simulink model "F16_fcs111"  (Simulink 9.1)
settings: Solver=ode3  StartTime=0.0  StopTime=simtime  FixedStep=0.001  RelTol=1e-3  EnableMultiTasking=on
values from neighbouring files (symbols this model uses):
  alpha_trim = xu(3)    [runF16fcs.m]
  dlef_trim = uu(5)    [runF16fcs.m]
  fi_flag_Simulink = 1    [runF16fcs.m]
  V_trim = xu(1)    [runF16fcs.m]
undefined symbols (not defined in the file or in its folder): Earth, m, s, WGS84
libraries: simulink_extras x6, aerolibconvert2 x2, sharedtransform x2, aerolibtransform2 x1, aerolibconvert x1, aerolibobsolete x1, aerolibanimutils x1
settings Model: SuppressorTable="22 serialization::archive 11 0 6 0 0 1 8 0 0 0 0 6 0 0 1 0 49 F16_fcs111/Display Results/cascvt/Unit Conversion 0 6 0 0 1 8 0 0 0 0 6 49 SimulinkFixedPoint:util:fxpParameterPrecisionLoss 0 0 0 6 0  11 Wenchao Lei 0 0 0 0 8 20180715 0 0 0 16 3 53 0 0"  Creator=larssonneveldt  LastModifiedBy=Wenchao Lei
settings DataIOCC: LimitDataPoints=on  SignalLoggingSaveFormat=ModelDataLogs  SignalLoggingName=sigsOut
settings OptimizationCC: ExpressionDepthLimit=2147483647  InitFltsAndDblsToZero=on
settings DebuggingCC: SignalResolutionControl=TryResolveAllWithWarning  MultiTaskDSMMsg=warning  MultiTaskCondExecSysMsg=none  ParameterPrecisionLossMsg=none  FcnCallInpInsideContextMsg=warning  StateNameClashWarn=warning
settings HardwareCC: TargetHWDeviceType=32-bit Generic  TargetUnknown=on  ProdEqTarget=off
settings GRTTargetCC: TargetFcnLib=ansi_tfl_tmw.mat

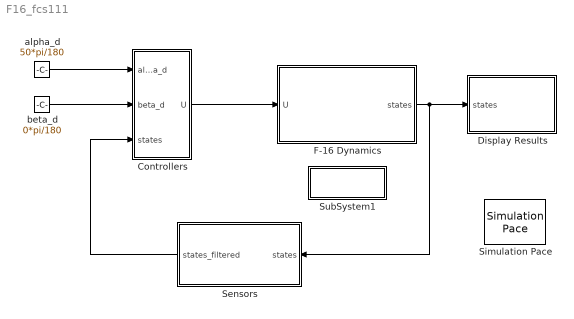
== system F16_fcs111 ==
  Controllers : Subsystem
  Display Results : Subsystem
  F-16 Dynamics : Subsystem
      mask Display: image(imread('aerodata/f16.jpg'))
  Sensors : Subsystem
  Simulation Pace : aerolibanimutils/Simulation Pace  SimulationPace=10  SleepMode=MATLAB Thread  OutputPaceError=off  SampleTime=-1
      settings: AttributesFormatString=%<SimulationPace> sec/sec
  SubSystem1 : Subsystem
      settings: OpenFcn=edit(fullfile(cd,'F16_dyn.c'))
      mask Display: disp('F16_dyn.c');
  alpha_d : Constant  Value=50*pi/180
  beta_d : Constant  Value=0*pi/180
  wires:
  F-16 Dynamics/1(states) -> Display Results/1(states), Sensors/1(states)
  Sensors/1(states_filtered) -> Controllers/3(states)
  beta_d/1 -> Controllers/2(beta_d)
  Controllers/1(U) -> F-16 Dynamics/1(U)
  alpha_d/1 -> Controllers/1(alpha_d)

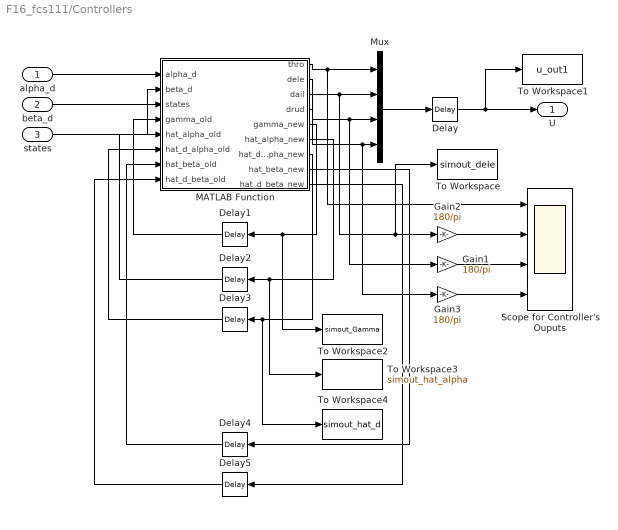
== system F16_fcs111/Controllers ==
  alpha_d : Inport
  beta_d : Inport  Port=2
  states : Inport  Port=3
  Delay : TransportDelay  DelayTime=0.02
  Delay1 : TransportDelay  DelayTime=0.01  InitialOutput=0.1*ones(3,1)
  Delay{2..5} (4 alike) : TransportDelay  DelayTime=0.01
  Gain1 : Gain  Gain=180/pi
  Gain2 : Gain  Gain=180/pi
  Gain3 : Gain  Gain=180/pi
  MATLAB Function : MATLAB Function  TreatAsAtomicUnit=on
  Mux : Mux
  Scope for Controller's Ouputs : Scope  NumInputPorts=4
  To Workspace : ToWorkspace  VariableName=simout_dele  SaveFormat=Structure With Time  SampleTime=-1
  To Workspace1 : ToWorkspace  VariableName=u_out1  SaveFormat=Structure With Time  SampleTime=-1
  To Workspace2 : ToWorkspace  VariableName=simout_Gamma  SaveFormat=Structure With Time  SampleTime=-1
  To Workspace3 : ToWorkspace  VariableName=simout_hat_alpha  SaveFormat=Structure With Time  SampleTime=-1
  To Workspace4 : ToWorkspace  VariableName=simout_hat_d  SaveFormat=Structure With Time  SampleTime=-1
  U : Outport
  wires:
  beta_d/1 -> MATLAB Function/2(beta_d)
  Mux/1 -> Delay/1
  Delay/1 -> U/1, To Workspace1/1
  states/1 -> MATLAB Function/3(states)
  alpha_d/1 -> MATLAB Function/1(alpha_d)
  Gain2/1 -> Scope for Controller's Ouputs/2
  Gain1/1 -> Scope for Controller's Ouputs/3
  Gain3/1 -> Scope for Controller's Ouputs/4
  Delay1/1 -> MATLAB Function/4(gamma_old)
  MATLAB Function/1(thro) -> Scope for Controller's Ouputs/1, Mux/1
  MATLAB Function/2(dele) -> To Workspace/1, Gain2/1, Mux/2
  MATLAB Function/3(dail) -> Gain1/1, Mux/3
  MATLAB Function/5(gamma_new) -> To Workspace2/1, Delay1/1
  MATLAB Function/4(drud) -> Gain3/1, Mux/4
  MATLAB Function/6(hat_alpha_new) -> To Workspace3/1, Delay2/1
  Delay2/1 -> MATLAB Function/5(hat_alpha_old)
  MATLAB Function/7(hat_d_alpha_new) -> To Workspace4/1, Delay3/1
  Delay3/1 -> MATLAB Function/6(hat_d_alpha_old)
  MATLAB Function/8(hat_beta_new) -> Delay4/1
  Delay4/1 -> MATLAB Function/7(hat_beta_old)
  MATLAB Function/9(hat_d_beta_new) -> Delay5/1
  Delay5/1 -> MATLAB Function/8(hat_d_beta_old)

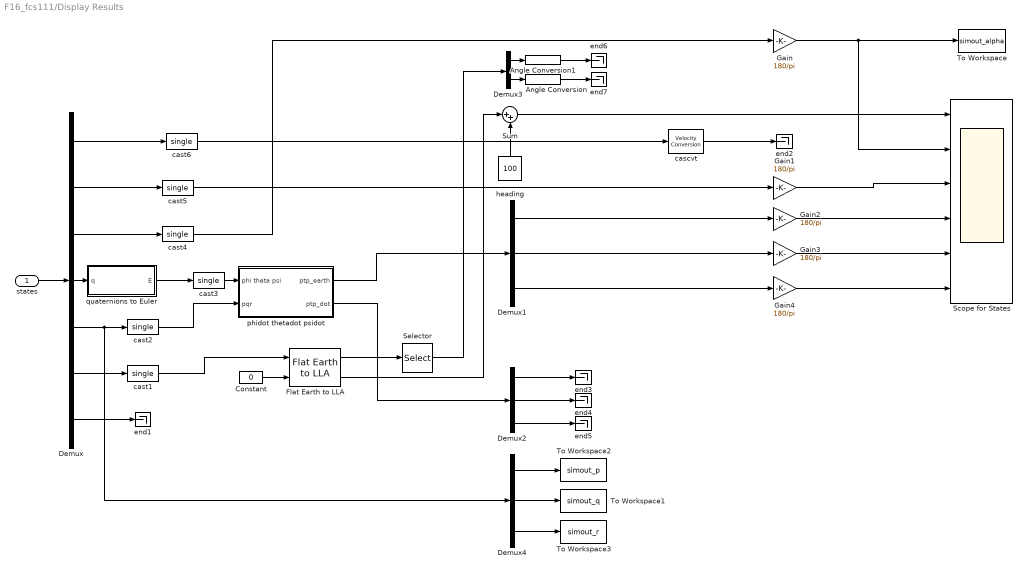
== system F16_fcs111/Display Results ==
  states : Inport
  Angle Conversion : aerolibconvert2/Angle Conversion  IU=deg  OU=rad
  Angle Conversion1 : aerolibconvert2/Angle Conversion  IU=deg  OU=rad
  Constant : Constant  Value=0
  Demux : Demux  Outputs=[1 1 1 4 3 3 3]
  Demux1 : Demux  Outputs=3
  Demux2 : Demux  Outputs=3
  Demux3 : Demux  Outputs=2
  Demux4 : Demux  Outputs=3
  Flat Earth to LLA : aerolibtransform2/Flat Earth to LLA  units=Metric (MKS)  ptype=Earth (WGS84)  F=1/298.257223563  R=6378137  LL0=[37.7889 -122.4778]  psi=0
  Gain{,1..4} (5 alike) : Gain  Gain=180/pi
  Scope for States : Scope  NumInputPorts=6
  Selector : Selector  InputPortWidth=2  IndexOptions=Index vector (dialog)  Indices=[2 1]  OutputSizes=1
  Sum : Sum  Inputs=|++
  To Workspace : ToWorkspace  VariableName=simout_alpha  SaveFormat=Structure With Time  SampleTime=-1
  To Workspace1 : ToWorkspace  VariableName=simout_q  SaveFormat=Structure With Time  SampleTime=-1
  To Workspace2 : ToWorkspace  VariableName=simout_p  SaveFormat=Structure With Time  SampleTime=-1
  To Workspace3 : ToWorkspace  VariableName=simout_r  SaveFormat=Structure With Time  SampleTime=-1
  cascvt : aerolibconvert/Velocity Conversion  IU=m/s  OU=kts
      settings: SourceProductName=Aerospace Blockset  SourceProductBaseCode=AE
  cast{1..6} (6 alike) : DataTypeConversion  OutDataTypeStr=single  SaturateOnIntegerOverflow=on
  end{1..7} (7 alike) : Terminator
  heading : Constant  Value=100
  phidot thetadot psidot : Subsystem
  quaternions to Euler : Subsystem
  wires:
  states/1 -> Demux/1
  Demux/1 -> cast6/1
  Demux/2 -> cast5/1
  Demux1/1 -> Gain2/1
  Demux1/3 -> Gain4/1
  Demux/3 -> cast4/1
  Demux/5 -> cast2/1, Demux4/1
  phidot thetadot psidot/1(ptp_earth) -> Demux1/1
  phidot thetadot psidot/2(ptp_dot) -> Demux2/1
  Demux/6 -> cast1/1
  Constant/1 -> Flat Earth to LLA/2
  Flat Earth to LLA/1 -> Selector/1
  Selector/1 -> Demux3/1
  Demux3/1 -> Angle Conversion1/1
  Demux3/2 -> Angle Conversion/1
  cast1/1 -> Flat Earth to LLA/1
  cast2/1 -> phidot thetadot psidot/2(pqr)
  cast3/1 -> phidot thetadot psidot/1(phi theta psi)
  cast4/1 -> Gain/1
  cast5/1 -> Gain1/1
  cast6/1 -> cascvt/1
  Flat Earth to LLA/2 -> Sum/1
  Sum/1 -> Scope for States/1
  heading/1 -> Sum/2
  quaternions to Euler/1(E) -> cast3/1
  Demux/4 -> quaternions to Euler/1(q)
  Demux/7 -> end1/1
  Gain3/1 -> Scope for States/5
  Gain2/1 -> Scope for States/4
  Gain4/1 -> Scope for States/6
  Demux1/2 -> Gain3/1
  Gain/1 -> Scope for States/2, To Workspace/1
  Gain1/1 -> Scope for States/3
  Demux4/1 -> To Workspace2/1
  Demux4/3 -> To Workspace3/1
  Demux4/2 -> To Workspace1/1
  cascvt/1 -> end2/1
  Demux2/1 -> end3/1
  Demux2/2 -> end4/1
  Demux2/3 -> end5/1
  Angle Conversion1/1 -> end6/1
  Angle Conversion/1 -> end7/1

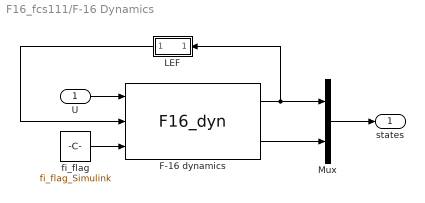
== system F16_fcs111/F-16 Dynamics ==
  U : Inport
  F-16 dynamics : S-Function  FunctionName=F16_dyn  Parameters=init_x  SFunctionDeploymentMode=off  EnableBusSupport=off
      mask Display: image(imread('aerodata/f16.jpg'))
  LEF : Subsystem
      mask Display: port_label('output', 1, 'dlef')
  Mux : Mux  Inputs=2
  fi_flag : Constant  Value=fi_flag_Simulink
  states : Outport
  wires:
  fi_flag/1 -> F-16 dynamics/3
  LEF/1("delta_lef ") -> F-16 dynamics/2
  U/1 -> F-16 dynamics/1
  F-16 dynamics/1 -> LEF/1(state), Mux/1
  F-16 dynamics/2 -> Mux/2
  Mux/1 -> states/1

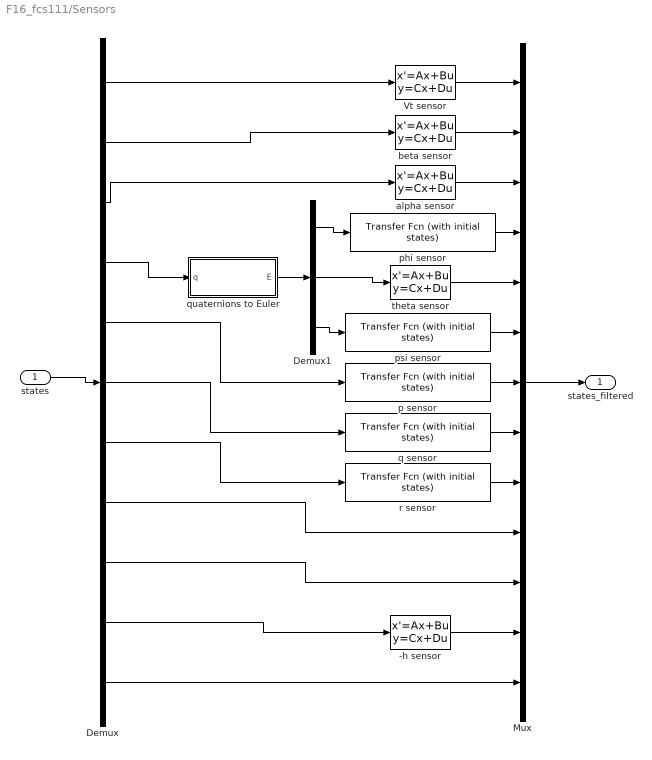
== system F16_fcs111/Sensors ==
  states : Inport
  -h sensor : StateSpace  A=-50  B=50  D=0  InitialCondition=alpha_trim
  Demux : Demux  Outputs=[ones(1,3) 4 ones(1,6) 3]
  Demux1 : Demux  Outputs=3
  Mux : Mux  Inputs=[ones(1,12) 3]
  Vt sensor : StateSpace  A=-50  B=50  D=0  InitialCondition=V_trim
  alpha sensor : StateSpace  A=-50  B=50  D=0  InitialCondition=alpha_trim
  beta sensor : StateSpace  A=-50  B=50  D=0  InitialCondition=0
  p sensor : simulink_extras/Additional Linear/Transfer Fcn (with initial states)  N=[0.0001903 0.005346 1]  D=[0.0004942 0.03082 1]  X0=[0 0]
  phi sensor : simulink_extras/Additional Linear/Transfer Fcn (with initial states)  N=[1]  D=[0.00104 0.0323 1]  X0=[0 0]
  psi sensor : simulink_extras/Additional Linear/Transfer Fcn (with initial states)  N=[1]  D=[0.00104 0.0323 1]  X0=[0 0]
  q sensor : simulink_extras/Additional Linear/Transfer Fcn (with initial states)  N=[0.0001903 0.005346 1]  D=[0.0004942 0.03082 1]  X0=[0 0]
  quaternions to Euler : Subsystem
  r sensor : simulink_extras/Additional Linear/Transfer Fcn (with initial states)  N=[0.0001903 0.005346 1]  D=[0.0004942 0.03082 1]  X0=[0 0]
  theta sensor : StateSpace  A=-50  B=50  D=0  InitialCondition=alpha_trim
  states_filtered : Outport
  wires:
  Mux/1 -> states_filtered/1
  states/1 -> Demux/1
  r sensor/1 -> Mux/9
  q sensor/1 -> Mux/8
  p sensor/1 -> Mux/7
  psi sensor/1 -> Mux/6
  phi sensor/1 -> Mux/4
  alpha sensor/1 -> Mux/3
  beta sensor/1 -> Mux/2
  Vt sensor/1 -> Mux/1
  Demux1/1 -> phi sensor/1
  Demux1/2 -> theta sensor/1
  Demux1/3 -> psi sensor/1
  -h sensor/1 -> Mux/12
  quaternions to Euler/1(E) -> Demux1/1
  theta sensor/1 -> Mux/5
  Demux/1 -> Vt sensor/1
  Demux/2 -> beta sensor/1
  Demux/3 -> alpha sensor/1
  Demux/4 -> quaternions to Euler/1(q)
  Demux/5 -> p sensor/1
  Demux/6 -> q sensor/1
  Demux/7 -> r sensor/1
  Demux/8 -> Mux/10
  Demux/9 -> Mux/11
  Demux/10 -> -h sensor/1
  Demux/11 -> Mux/13

== system F16_fcs111/SubSystem1 ==

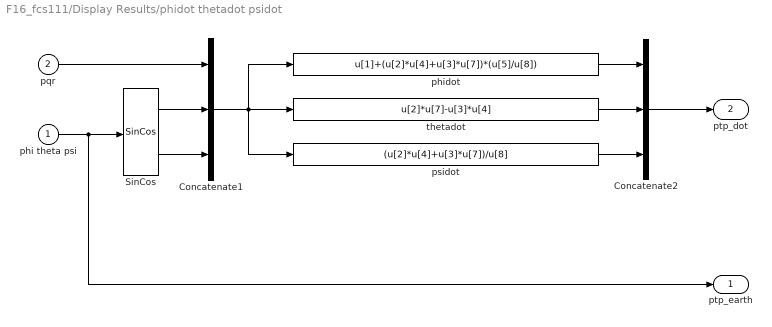
== system F16_fcs111/Display Results/phidot thetadot psidot ==
  phi theta psi : Inport
  pqr : Inport  Port=2
  Concatenate1 : Concatenate  NumInputs=3
  Concatenate2 : Concatenate  NumInputs=3
  SinCos : aerolibobsolete/SinCos
      settings: SourceProductName=Aerospace Blockset  SourceProductBaseCode=AE
  phidot : Fcn  Expr=u[1]+(u[2]*u[4]+u[3]*u[7])*(u[5]/u[8])
  psidot : Fcn  Expr=(u[2]*u[4]+u[3]*u[7])/u[8]
  thetadot : Fcn  Expr=u[2]*u[7]-u[3]*u[4]
  ptp_earth : Outport
  ptp_dot : Outport  Port=2
  wires:
  Concatenate1/1 -> psidot/1, phidot/1, thetadot/1
  pqr/1 -> Concatenate1/1
  phi theta psi/1 -> SinCos/1, ptp_earth/1
  psidot/1 -> Concatenate2/3
  thetadot/1 -> Concatenate2/2
  phidot/1 -> Concatenate2/1
  Concatenate2/1 -> ptp_dot/1
  SinCos/1 -> Concatenate1/2
  SinCos/2 -> Concatenate1/3

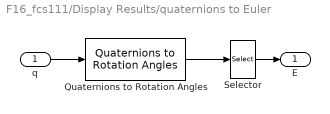
== system F16_fcs111/Display Results/quaternions to Euler ==
  q : Inport
  Quaternions to Rotation Angles : sharedtransform/Quaternions to Rotation Angles  rotationOrder=ZYX  aMode=aMode
      settings: SourceProductBaseCode=AE
  Selector : Selector  InputPortWidth=3  IndexOptions=Index vector (dialog)  Indices=[3 2 1]  OutputSizes=1
  E : Outport
  wires:
  Quaternions to Rotation Angles/1 -> Selector/1
  q/1 -> Quaternions to Rotation Angles/1
  Selector/1 -> E/1

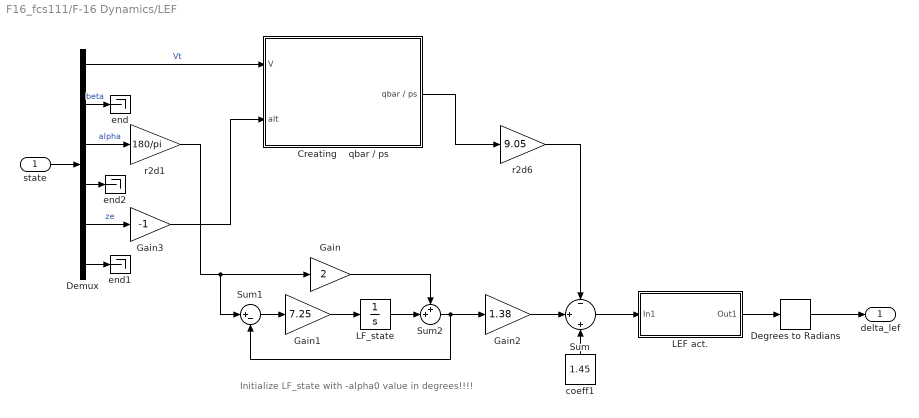
== system F16_fcs111/F-16 Dynamics/LEF ==
  note: Initialize LF_state with -alpha0 value in degrees!!!!
  state : Inport
  Creating    qbar / ps : Subsystem
  Degrees to Radians : simulink_extras/Transformations/Degrees to Radians
  Demux : Demux  Outputs=[1 1 1 9 1 1]
  Gain : Gain  Gain=2  SaturateOnIntegerOverflow=on  OutDataTypeStr=Inherit: Same as input  ParamDataTypeStr=Inherit: Same as input
  Gain1 : Gain  Gain=7.25  SaturateOnIntegerOverflow=on  OutDataTypeStr=Inherit: Same as input  ParamDataTypeStr=Inherit: Same as input
  Gain2 : Gain  Gain=1.38  SaturateOnIntegerOverflow=on  OutDataTypeStr=Inherit: Same as input  ParamDataTypeStr=Inherit: Same as input
  Gain3 : Gain  Gain=-1  SaturateOnIntegerOverflow=on  OutDataTypeStr=Inherit: Same as input  ParamDataTypeStr=Inherit: Same as input
  LEF act. : Subsystem
  LF_state : Integrator  InitialCondition=-alpha_trim*180/pi
  Sum : Sum  Inputs=-|+|+  SaturateOnIntegerOverflow=on  InputSameDT=on  OutDataTypeStr=Inherit: Same as first input
  Sum1 : Sum  Inputs=|+-  SaturateOnIntegerOverflow=on  InputSameDT=on  OutDataTypeStr=Inherit: Same as first input
  Sum2 : Sum  Inputs=++|  SaturateOnIntegerOverflow=on  InputSameDT=on  OutDataTypeStr=Inherit: Same as first input
  coeff1 : Constant  Value=1.45
  end : Terminator
  end1 : Terminator
  end2 : Terminator
  r2d1 : Gain  Gain=180/pi  SaturateOnIntegerOverflow=on  OutDataTypeStr=Inherit: Same as input  ParamDataTypeStr=Inherit: Same as input
  r2d6 : Gain  Gain=9.05  SaturateOnIntegerOverflow=on  OutDataTypeStr=Inherit: Same as input  ParamDataTypeStr=Inherit: Same as input
  "delta_lef " : Outport
  wires:
  Degrees to Radians/1 -> "delta_lef "/1
  Gain3/1 -> Creating    qbar / ps/2(alt)
  LEF act./1(Out1) -> Degrees to Radians/1
  Sum/1 -> LEF act./1(In1)
  state/1 -> Demux/1
  Sum1/1 -> Gain1/1
  Gain1/1 -> LF_state/1
  Gain/1 -> Sum2/1
  Gain2/1 -> Sum/2
  coeff1/1 -> Sum/3
  Sum2/1 -> Sum1/2, Gain2/1
  LF_state/1 -> Sum2/2
  r2d1/1 -> Sum1/1, Gain/1
  Creating    qbar / ps/1(qbar / ps) -> r2d6/1
  r2d6/1 -> Sum/1
  Demux/1 -> Creating    qbar / ps/1(V)  "Vt"
  Demux/2 -> end/1  "beta"
  Demux/3 -> r2d1/1  "alpha"
  Demux/4 -> end2/1
  Demux/5 -> Gain3/1  "ze"
  Demux/6 -> end1/1

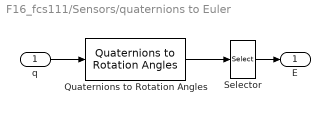
== system F16_fcs111/Sensors/quaternions to Euler ==
  q : Inport
  Quaternions to Rotation Angles : sharedtransform/Quaternions to Rotation Angles  rotationOrder=ZYX  aMode=aMode
      settings: SourceProductBaseCode=AE
  Selector : Selector  InputPortWidth=3  IndexOptions=Index vector (dialog)  Indices=[3 2 1]  OutputSizes=1
  E : Outport
  wires:
  Quaternions to Rotation Angles/1 -> Selector/1
  q/1 -> Quaternions to Rotation Angles/1
  Selector/1 -> E/1

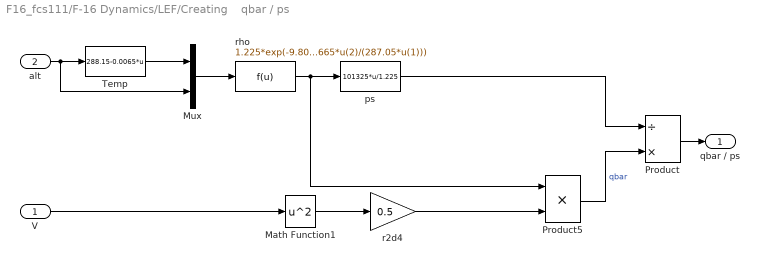
== system F16_fcs111/F-16 Dynamics/LEF/Creating    qbar / ps ==
  V : Inport
  alt : Inport  Port=2
  Math Function1 : Math  Operator=square  SaturateOnIntegerOverflow=on
  Mux : Mux  Inputs=2
  Product : Product  Inputs=/*  SaturateOnIntegerOverflow=on  InputSameDT=on  OutDataTypeStr=Inherit: Same as first input
  Product5 : Product  Inputs=**  SaturateOnIntegerOverflow=on  InputSameDT=on  OutDataTypeStr=Inherit: Same as first input
  Temp : Fcn  Expr=288.15-0.0065*u
  ps : Fcn  Expr=101325*u/1.225
  r2d4 : Gain  Gain=0.5  SaturateOnIntegerOverflow=on  OutDataTypeStr=Inherit: Same as input  ParamDataTypeStr=Inherit: Same as input
  rho : Fcn  Expr=1.225*exp(-9.80665*u(2)/(287.05*u(1)))
  qbar / ps : Outport
  wires:
  ps/1 -> Product/1
  rho/1 -> Product5/1, ps/1
  Mux/1 -> rho/1
  Temp/1 -> Mux/1
  alt/1 -> Mux/2, Temp/1
  Math Function1/1 -> r2d4/1
  r2d4/1 -> Product5/2
  Product5/1 -> Product/2  "qbar"
  Product/1 -> qbar / ps/1
  V/1 -> Math Function1/1

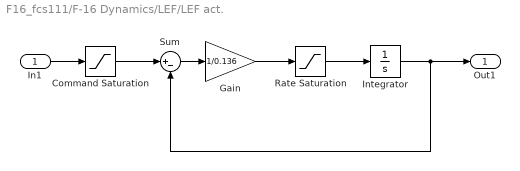
== system F16_fcs111/F-16 Dynamics/LEF/LEF act. ==
  In1 : Inport
  Command Saturation : Saturate  UpperLimit=25  LowerLimit=0
  Gain : Gain  Gain=1/0.136  SaturateOnIntegerOverflow=on  OutDataTypeStr=Inherit: Same as input  ParamDataTypeStr=Inherit: Same as input
  "Integrator " : Integrator  InitialCondition=dlef_trim*180/pi  UpperSaturationLimit=25  LowerSaturationLimit=-25
  Rate Saturation : Saturate  UpperLimit=25  LowerLimit=-25
  Sum : Sum  Inputs=|+-  SaturateOnIntegerOverflow=on  InputSameDT=on  OutDataTypeStr=Inherit: Same as first input
  Out1 : Outport
  wires:
  "Integrator "/1 -> Sum/2, Out1/1
  Rate Saturation/1 -> "Integrator "/1
  Gain/1 -> Rate Saturation/1
  Sum/1 -> Gain/1
  Command Saturation/1 -> Sum/1
  In1/1 -> Command Saturation/1

== matlab function Controllers/MATLAB Function ==
  data: alpha_d input double; beta_d input double; states input double; gamma_old input double; thro output double; dele output double; dail output double; drud output double; gamma_new output double; hat_alpha_old input double; hat_d_alpha_old input double; hat_alpha_new output double; hat_d_alpha_new output double; hat_beta_new output double; hat_d_beta_new output double; hat_beta_old input double; hat_d_beta_old input double
function [thro,dele,dail,drud, gamma_new, hat_alpha_new, hat_d_alpha_new, hat_beta_new, hat_d_beta_new] = Controller(alpha_d,beta_d,states, gamma_old, hat_alpha_old, hat_d_alpha_old,hat_beta_old,hat_d_beta_old)

h_sample = 0.01;
gamma_new = zeros(3,1);

k_alpha = 3.5;
k_q = 7;

k_beta = 2;
k_r = 4;

Ixx = 12874.8;
Iyy = 75673.6;
Izz = 85552.1;
Ixz = 1331.4;
Gamma = Ixx * Izz - (Ixz  * Ixz);
C1 = ((Iyy - Izz)  * Izz  - (Ixz * Ixz))/ Gamma;
C2 = ((Ixx - Iyy + Izz ) * Ixz ) / Gamma;
C3 = Izz / Gamma;
C4 = Ixz / Gamma;
C5 = (Izz - Ixx) / Iyy;
C6 = Ixz / Iyy ;
C7 = 1 / Iyy;
C8 = (Ixx * (Ixx - Iyy ) + Ixz * Ixz) / Gamma;
C9 = Ixx / Gamma;
Sref = 27.87;
bref = 9.144;
cref = 3.45;

vt = states(1);
beta = states(2);
alpha = states(3);
phi = states(4);
theta = states(5);
psi = states(6);
p = states(7);
q = states(8);
r = states(9);
x_earth = states(10);
y_earth = states(11);
z_earth = states(12);
power = states(13);
ny = states(14);
nz = states(15);

%% Dynamic Pressure
%%
rho0 = 1.22505;
Re = 6371000.0;
R = 287.04;
g0 = 9.80665;
pres0 = 101325.0;
temp0 = 288.16;
gamma = 1.403;
grad = -0.0065;

alt = -z_earth;

temp = temp0 + grad * alt;
pres = pres0*( (temp/temp0)^(-g0/(R*grad)) );
rho  = pres/(R*temp);

if (alt >= 11000.0)
    temp = temp0 + grad * 11000;
    pres  = pres0*( (temp/temp0)^(-g0/(R*grad)) )*10.0^(-g0*(alt-11000)/(2.3026*R*temp));
    rho   = pres0*( (temp/temp0)^(-g0/(R*grad)) )/(R*temp)*10.0^(-g0*(alt-11000)/(2.3026*R*temp));
end

mach = vt / sqrt(gamma * R * temp);
qbar = 0.5 * rho * vt * vt;
grav = g0*(Re*Re/((Re+alt)*(Re+alt)));

%% 
%%%%%%%%%%%%%%%%%%%%%%%%%%%%%%%%%%%%%%%%%%%%%%%%%%%%%%%%%%%
% Throttle
%%%%%%%%%%%%%%%%%%%%%%%%%%%%%%%%%%%%%%%%%%%%%%%%%%%%%%%%%%%
thro = 0;

%%
%%%%%%%%%%%%%%%%%%%%%%%%%%%%%%%%%%%%%%%%%%%%%%%%%%%%%%%%%%%
% AOA
%%%%%%%%%%%%%%%%%%%%%%%%%%%%%%%%%%%%%%%%%%%%%%%%%%%%%%%%%%%

%% ADRC Method
% ESO
pole_eso = 2;
k_eso_1 = 2*pole_eso;
k_eso_2 = pole_eso*pole_eso;
hat_alpha_new = hat_alpha_old + h_sample*( q + hat_d_alpha_old - k_eso_1*( hat_alpha_old - alpha) );
hat_d_alpha_new = hat_d_alpha_old + h_sample*( -k_eso_2*(hat_alpha_old - alpha) );


%% Outer Loop
%%
dalpha_d = 0;
e_alpha = alpha - alpha_d;
%q_ref = dalpha_d + (p*cos(alpha)+r*sin(alpha))*tan(beta) - k_alpha*e_alpha;
q_ref = dalpha_d - hat_d_alpha_new + 0*(p*cos(alpha)+r*sin(alpha))*tan(beta) - k_alpha*e_alpha;

%% Inner Loop
%%
e_q = q-q_ref;

%% PID Control Method
%% P
%drud_deg = ( -C5*p*r+C6*(p^2-r^2)-k_q*e_q )/(-C7*qbar*Sref*cref);

% Controller

%% Sliding Mode Control Method
%% CSMC
% Phi = 0.0085;
% if abs(e_q)<Phi
%     drud_deg = ( -C5*p*r+C6*(p^2-r^2)- 10*e_q/Phi )/(-C7*qbar*Sref*cref);
% else
%     drud_deg = ( -C5*p*r+C6*(p^2-r^2)- 10*sign(e_q) )/(-C7*qbar*Sref*cref);
% end
%% ASMC
% h_sample = 0.02;
% gamma_new(1) = gamma_old(1) + h_sample*2*e_q*sign(e_q); 
% drud_deg = ( -C5*p*r+C6*(p^2-r^2)- gamma_new(1)*sign(e_q) )/(-C7*qbar*Sref*cref);
%% AQSMC
mu = 30;
e_q_sigmoid = ( 1-exp(-mu*e_q) ) / ( 1+exp(-mu*e_q) );
h_sample = 0.02;
gamma_new(1) = gamma_old(1) + h_sample*2*e_q*e_q_sigmoid; 
drud_deg = ( -C5*p*r+C6*(p^2-r^2)- gamma_new(1)*e_q_sigmoid )/(-C7*qbar*Sref*cref);
%% Saturation
dele = drud_deg*pi/180*100*10/7*5/7/10*0.6;
dele = min(max(dele,-25*pi/180),25*pi/180);

%% 
%%%%%%%%%%%%%%%%%%%%%%%%%%%%%%%%%%%%%%%%%%%%%%%%%%%%%%%%%%%
% Roll
%%%%%%%%%%%%%%%%%%%%%%%%%%%%%%%%%%%%%%%%%%%%%%%%%%%%%%%%%%%
%% ADRC Method
% ESO
pole_eso = 2;
k_eso_1 = 2*pole_eso;
k_eso_2 = pole_eso*pole_eso;
hat_beta_new = hat_beta_old + h_sample*( p*sin(alpha) - r*cos(alpha) + hat_d_beta_old - k_eso_1*( hat_beta_old - beta) );
hat_d_beta_new = hat_d_beta_old + h_sample*( -k_eso_2*(hat_beta_old - beta) );

%% Outer Loop
%%
dbeta_d = 0;
e_beta = beta - beta_d ;
%r_ref = ( dbeta_d -p*sin(alpha) - k_beta*e_beta )/(-1*max(cos(alpha),1));%/(-cos(alpha));
r_ref = ( dbeta_d -p*sin(alpha) - hat_d_beta_new - k_beta*e_beta )/(-cos(alpha));%(-1*max(cos(alpha),1));%/(-cos(alpha));

%% Inner Loop
%%
e_r = r-r_ref;
%dail_deg = ( -(C8*p-C2*r)*q-k_r*e_r )/(-C4*qbar*Sref*bref);
%dail_deg = ( -(C8*p-C2*r)*q-sign(e_r) )/(-C4*qbar*Sref*bref);
mu = 40;
e_r_sigmoid = ( 1-exp(-mu*e_r) ) / ( 1+exp(-mu*e_r) );
gamma_new(2) = gamma_old(2) + h_sample*2*e_r*e_r_sigmoid; 
dail_deg = ( -(C8*p-C2*r)*q - gamma_new(2)*e_r_sigmoid )/(C4*qbar*Sref*bref);
dail = dail_deg*pi/180*100*10/7*5/7*20/5/5;

%% 
%%%%%%%%%%%%%%%%%%%%%%%%%%%%%%%%%%%%%%%%%%%%%%%%%%%%%%%%%%%
% AOS
%%%%%%%%%%%%%%%%%%%%%%%%%%%%%%%%%%%%%%%%%%%%%%%%%%%%%%%%%%%
%% Outer Loop
%%
dbeta_d = 0;
e_beta = beta - beta_d ;
%r_ref = ( dbeta_d -p*sin(alpha) - k_beta*e_beta )/(-1*max(cos(alpha),1));%/(-cos(alpha));
r_ref = ( dbeta_d -p*sin(alpha) - hat_d_beta_new - k_beta*e_beta )/(-cos(alpha));%(-1*max(cos(alpha),1));%/(-cos(alpha));

%% Inner Loop
%%
e_r = r-r_ref;
%drud_deg = ( -(C8*p-C2*r)*q-k_r*e_r )/(-C9*qbar*Sref*bref);
%drud_deg = ( -(C8*p-C2*r)*q-sign(e_r) )/(-C9*qbar*Sref*bref);
mu = 40;
e_r_sigmoid = ( 1-exp(-mu*e_r) ) / ( 1+exp(-mu*e_r) );
h_sample = 0.02;
gamma_new(3) = gamma_old(3) + h_sample*2*e_r*e_r_sigmoid; 
drud_deg = ( -(C8*p-C2*r)*q - gamma_new(3)*e_r_sigmoid )/(-C9*qbar*Sref*bref);
drud = drud_deg*pi/180*100*10/7*5/7*20/5;
